simulink model "ClosedLoop_Test"  (R2023b)
settings: Solver=VariableStepAuto  StartTime=0.0  StopTime=10.0  RelTol=1e-3
libraries: cstblocks x5
settings Model: Creator=PierluigiMeneses  LastModifiedBy=PierluigiMeneses

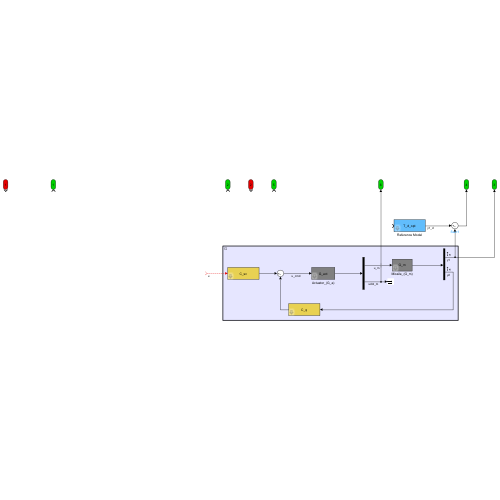
[thumbnail: Simulink's stored preview of the top-level diagram]
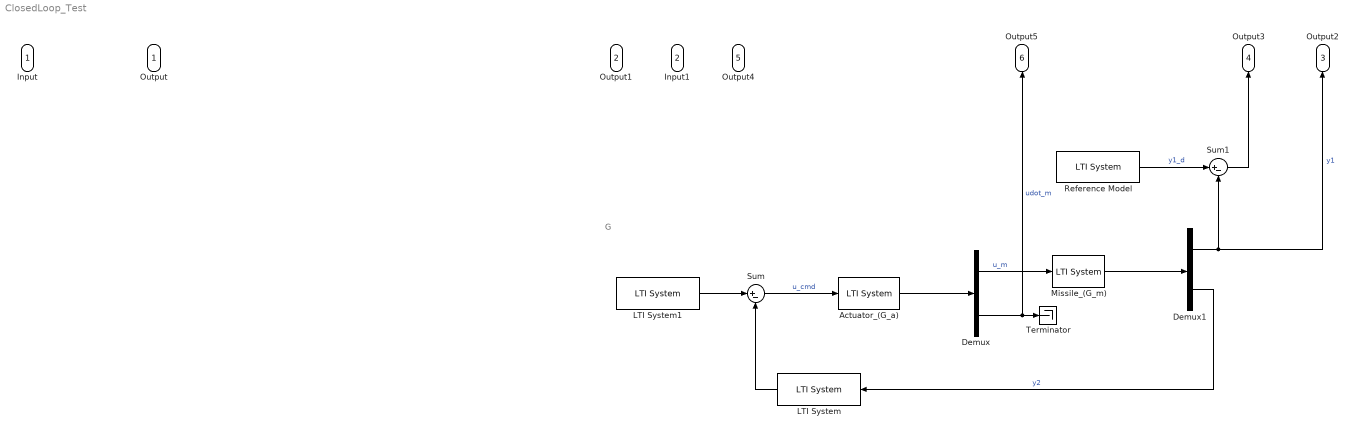
== system ClosedLoop_Test ==
  note: G
  Input : Inport
  Input1 : Inport  Port=2
  Actuator_(G_a) : cstblocks/LTI System  sys=G_act  IC=[]  PadeOrder=0
  Demux : Demux  Outputs=2
  Demux1 : Demux  Outputs=2
  LTI System : cstblocks/LTI System  sys=C_q  IC=[]  PadeOrder=0
  LTI System1 : cstblocks/LTI System  sys=C_sc  IC=[]  PadeOrder=0
  Missile_(G_m) : cstblocks/LTI System  sys=G_m  IC=[]  PadeOrder=0
  Reference Model : cstblocks/LTI System  sys=T_d_opt  IC=[]  PadeOrder=0
  Sum : Sum  Inputs=|+-
  Sum1 : Sum  Inputs=|+-
  Terminator : Terminator
  Output : Outport
  Output1 : Outport  Port=2
  Output2 : Outport  Port=3
  Output3 : Outport  Port=4
  Output4 : Outport  Port=5
  Output5 : Outport  Port=6
  wires:
  ? -> LTI System1/1  "u"
  Demux/1 -> Missile_(G_m)/1  "u_m"
  Demux1/2 -> LTI System/1  "y2"
  LTI System1/1 -> Sum/1
  Actuator_(G_a)/1 -> Demux/1
  Missile_(G_m)/1 -> Demux1/1
  Sum/1 -> Actuator_(G_a)/1  "u_cmd"
  LTI System/1 -> Sum/2
  Demux/2 -> Output5/1, Terminator/1  "udot_m"
  Reference Model/1 -> Sum1/1  "y1_d"
  Sum1/1 -> Output3/1
  Demux1/1 -> Output2/1, Sum1/2  "y1"
